simulink model "Model1"  (R2017a)
settings: Solver=ode23  StartTime=0.0  StopTime=10.0  RelTol=1e-8
values from neighbouring files (symbols this model uses):
  param = evalin('base','param')    [getSaveInfo.m]    (also in loadBackUp.m)
  u1 = 5    [Debug1.m]    (also in Model1Debug.m = 1)
  u2 = 0    [Debug1.m]    (also in Model1Debug.m)
  u3 = 0    [Debug1.m]    (also in Model1Debug.m)
  u4 = 0    [Debug1.m]    (also in Model1Debug.m = 3.25)
  u5 = 0    [Debug1.m]    (also in Model1Debug.m)
(part 1 of 3)
settings Model: Creator=www  LastModifiedBy=www
settings SolverCC: MaxConsecutiveMinStep=1000  ShapePreserveControl=EnableAll  ZeroCrossAlgorithm=Adaptive
settings DataIOCC: SaveOutput=off  SignalLogging=off  DSMLogging=off  SaveTime=off

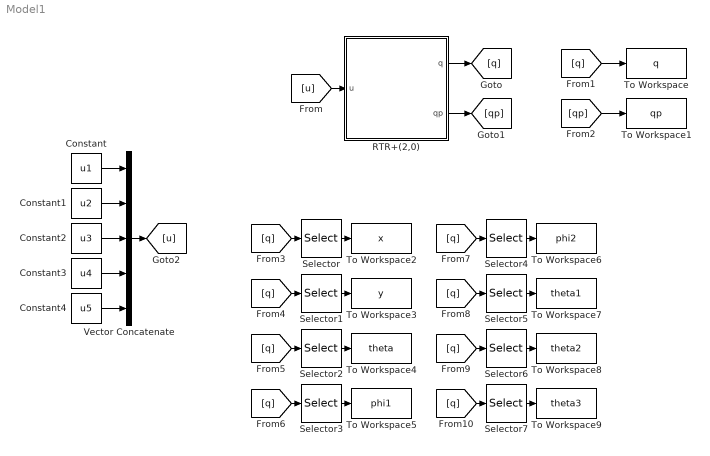
== system Model1 ==
  Constant : Constant  Value=u1
  Constant1 : Constant  Value=u2
  Constant2 : Constant  Value=u3
  Constant3 : Constant  Value=u4
  Constant4 : Constant  Value=u5
  RTR+(2,0) : Subsystem
  Selector : Selector  InputPortWidth=8  IndexOptions=Index vector (dialog)  Indices=1  OutputSizes=1
  Selector1 : Selector  InputPortWidth=8  IndexOptions=Index vector (dialog)  Indices=2  OutputSizes=1
  Selector2 : Selector  InputPortWidth=8  IndexOptions=Index vector (dialog)  Indices=3  OutputSizes=1
  Selector3 : Selector  InputPortWidth=8  IndexOptions=Index vector (dialog)  Indices=4  OutputSizes=1
  Selector4 : Selector  InputPortWidth=8  IndexOptions=Index vector (dialog)  Indices=5  OutputSizes=1
  Selector5 : Selector  InputPortWidth=8  IndexOptions=Index vector (dialog)  Indices=6  OutputSizes=1
  Selector6 : Selector  InputPortWidth=8  IndexOptions=Index vector (dialog)  Indices=7  OutputSizes=1
  Selector7 : Selector  InputPortWidth=8  IndexOptions=Index vector (dialog)  Indices=8  OutputSizes=1
  To Workspace : ToWorkspace  VariableName=q  SaveFormat=Timeseries  SampleTime=-1
  To Workspace1 : ToWorkspace  VariableName=qp  SaveFormat=Timeseries  SampleTime=-1
  To Workspace2 : ToWorkspace  VariableName=x  SampleTime=-1
  To Workspace3 : ToWorkspace  VariableName=y  SampleTime=-1
  To Workspace4 : ToWorkspace  VariableName=theta  SaveFormat=Timeseries  SampleTime=-1
  To Workspace5 : ToWorkspace  VariableName=phi1  SaveFormat=Timeseries  SampleTime=-1
  To Workspace6 : ToWorkspace  VariableName=phi2  SaveFormat=Timeseries  SampleTime=-1
  To Workspace7 : ToWorkspace  VariableName=theta1  SaveFormat=Timeseries  SampleTime=-1
  To Workspace8 : ToWorkspace  VariableName=theta2  SaveFormat=Timeseries  SampleTime=-1
  To Workspace9 : ToWorkspace  VariableName=theta3  SaveFormat=Timeseries  SampleTime=-1
  Vector Concatenate : Concatenate  NumInputs=5
  wires:
  Constant/1 -> Vector Concatenate/1
  Constant1/1 -> Vector Concatenate/2
  Constant4/1 -> Vector Concatenate/5
  Constant3/1 -> Vector Concatenate/4
  Constant2/1 -> Vector Concatenate/3
  RTR+(2,0)/1(q) -> [q]
  RTR+(2,0)/2(qp) -> [qp]
  [u] -> RTR+(2,0)/1(u)
  Vector Concatenate/1 -> [u]
  [q] -> To Workspace/1
  [qp] -> To Workspace1/1
  Selector/1 -> To Workspace2/1
  [q] -> Selector/1
  Selector1/1 -> To Workspace3/1
  [q] -> Selector1/1
  Selector2/1 -> To Workspace4/1
  [q] -> Selector2/1
  Selector3/1 -> To Workspace5/1
  [q] -> Selector3/1
  Selector4/1 -> To Workspace6/1
  [q] -> Selector4/1
  Selector5/1 -> To Workspace7/1
  [q] -> Selector5/1
  Selector6/1 -> To Workspace8/1
  [q] -> Selector6/1
  Selector7/1 -> To Workspace9/1
  [q] -> Selector7/1

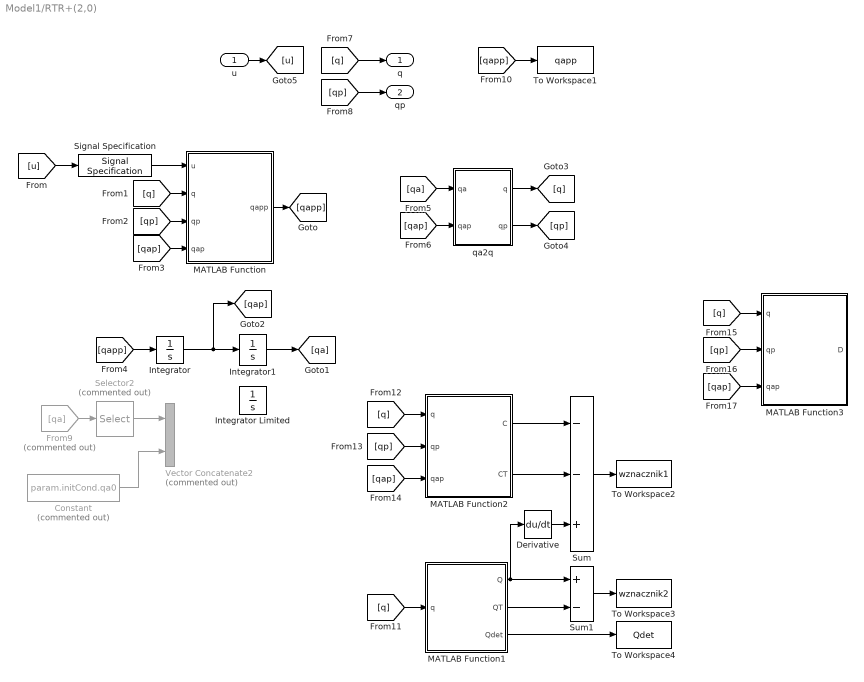
== system Model1/RTR+(2,0) ==
  u : Inport
  Constant : Constant  Commented=on  Value=param.initCond.qa0
  Derivative : Derivative
  From9 : From  Commented=on  GotoTag=qa
  Integrator : Integrator  InitialCondition=param.initCond.qap0
  Integrator Limited : Integrator  InitialCondition=param.initCond.qa0  LimitOutput=on  UpperSaturationLimit=50  LowerSaturationLimit=-50
  Integrator1 : Integrator  InitialCondition=param.initCond.qa0
  MATLAB Function : MATLAB Function  TreatAsAtomicUnit=on
  MATLAB Function1 : MATLAB Function  TreatAsAtomicUnit=on
  MATLAB Function2 : MATLAB Function  TreatAsAtomicUnit=on
  MATLAB Function3 : MATLAB Function  TreatAsAtomicUnit=on
  Selector2 : Selector  Commented=on  InputPortWidth=5  IndexOptions=Index vector (dialog)  Indices=[1 2]  OutputSizes=1
  Signal Specification : SignalSpecification  Dimensions=[5 1]
  Sum : Sum  Inputs=--+
  Sum1 : Sum  Inputs=+-
  To Workspace1 : ToWorkspace  VariableName=qapp  SaveFormat=Timeseries  SampleTime=-1
  To Workspace2 : ToWorkspace  VariableName=wznacznik1  SaveFormat=Timeseries  SampleTime=-1
  To Workspace3 : ToWorkspace  VariableName=wznacznik2  SaveFormat=Timeseries  SampleTime=-1
  To Workspace4 : ToWorkspace  VariableName=Qdet  SaveFormat=Timeseries  SampleTime=-1
  Vector Concatenate2 : Concatenate  Commented=on
  qa2q : Subsystem
  q : Outport
  qp : Outport  Port=2
  wires:
  [qp] -> MATLAB Function/3(qp)
  u/1 -> [u]
  MATLAB Function/1(qapp) -> [qapp]
  [qa] -> qa2q/1(qa)
  qa2q/2(qp) -> [qp]
  [u] -> Signal Specification/1
  [qp] -> qp/1
  qa2q/1(q) -> [q]
  [qap] -> qa2q/2(qap)
  [qap] -> MATLAB Function/4(qap)
  [qapp] -> Integrator/1
  [q] -> q/1
  [q] -> MATLAB Function/2(q)
  Integrator/1 -> Integrator1/1, [qap]
  Signal Specification/1 -> MATLAB Function/1(u)
  Constant/1 -> Vector Concatenate2/2
  Selector2/1 -> Vector Concatenate2/1
  From9/1 -> Selector2/1
  Integrator1/1 -> [qa]
  [qapp] -> To Workspace1/1
  [q] -> MATLAB Function1/1(q)
  MATLAB Function1/3(Qdet) -> To Workspace4/1
  [q] -> MATLAB Function2/1(q)
  [qp] -> MATLAB Function2/2(qp)
  [qap] -> MATLAB Function2/3(qap)
  [qap] -> MATLAB Function3/3(qap)
  [q] -> MATLAB Function3/1(q)
  [qp] -> MATLAB Function3/2(qp)
  Sum/1 -> To Workspace2/1
  MATLAB Function1/2(QT) -> Sum1/2
  Sum1/1 -> To Workspace3/1
  MATLAB Function2/1(C) -> Sum/1
  MATLAB Function2/2(CT) -> Sum/2
  Derivative/1 -> Sum/3
  MATLAB Function1/1(Q) -> Derivative/1, Sum1/1

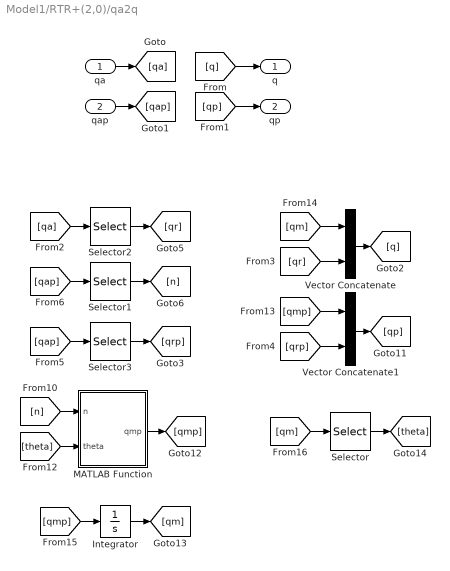
== system Model1/RTR+(2,0)/qa2q ==
  qa : Inport
  qap : Inport  Port=2
  Integrator : Integrator  InitialCondition=param.initCond.qm0
  MATLAB Function : MATLAB Function  TreatAsAtomicUnit=on
  Selector : Selector  InputPortWidth=5  IndexOptions=Index vector (dialog)  Indices=[3]  OutputSizes=1
  Selector1 : Selector  InputPortWidth=5  IndexOptions=Index vector (dialog)  Indices=[1 2]  OutputSizes=1
  Selector2 : Selector  InputPortWidth=5  IndexOptions=Index vector (dialog)  Indices=[3 4 5]  OutputSizes=1
  Selector3 : Selector  InputPortWidth=5  IndexOptions=Index vector (dialog)  Indices=[3 4 5]  OutputSizes=1
  Vector Concatenate : Concatenate
  Vector Concatenate1 : Concatenate
  q : Outport
  qp : Outport  Port=2
  wires:
  qa/1 -> [qa]
  qap/1 -> [qap]
  [q] -> q/1
  [qp] -> qp/1
  [qa] -> Selector2/1
  Vector Concatenate/1 -> [q]
  [qap] -> Selector1/1
  Vector Concatenate1/1 -> [qp]
  [n] -> MATLAB Function/1(n)
  [theta] -> MATLAB Function/2(theta)
  MATLAB Function/1(qmp) -> [qmp]
  [qmp] -> Vector Concatenate1/1
  [qm] -> Vector Concatenate/1
  Integrator/1 -> [qm]
  [qmp] -> Integrator/1
  [qm] -> Selector/1
  Selector/1 -> [theta]
  Selector1/1 -> [n]
  [qr] -> Vector Concatenate/2
  [qrp] -> Vector Concatenate1/2
  Selector2/1 -> [qr]
  Selector3/1 -> [qrp]
  [qap] -> Selector3/1

== matlab function Model1/RTR+(2,0)/qa2q/MATLAB Function ==
  data: n input; qmp output; theta input
function qmp = fcn(n,theta)
L=0.3;
R=0.075;
qmp=[cos(theta), cos(theta);
    sin(theta), sin(theta)
    1/L, -1/L;
    2/R, 0;
    0, 2/R]*n;
